simulink model "SMC_David_RedondoQuintero"  (R2023b)
settings: Solver=ode45  StartTime=0.0  StopTime=50  MaxStep=0.01  RelTol=1e-3
InitFcn:
  | R=2;
  | L=0.5;
  | Kb=0.01;
  | Ke=0.5;
  | Kt=0.5;
  | J=0.05;
undefined symbols (not defined in the file): sgn
libraries: simulink x3
settings Model: Creator=Usuario  LastModifiedBy=Usuario
settings SolverCC: ZeroCrossAlgorithm=Adaptive

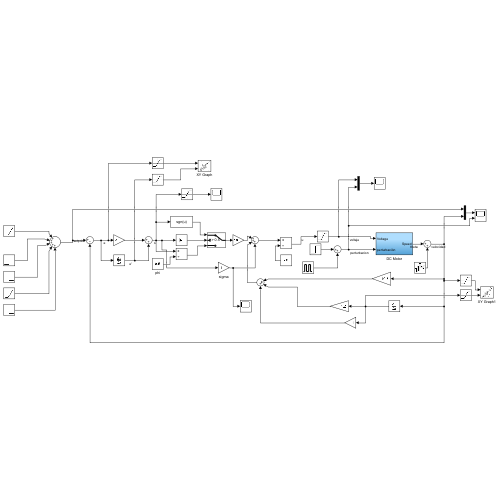
[thumbnail: Simulink's stored preview of the top-level diagram]
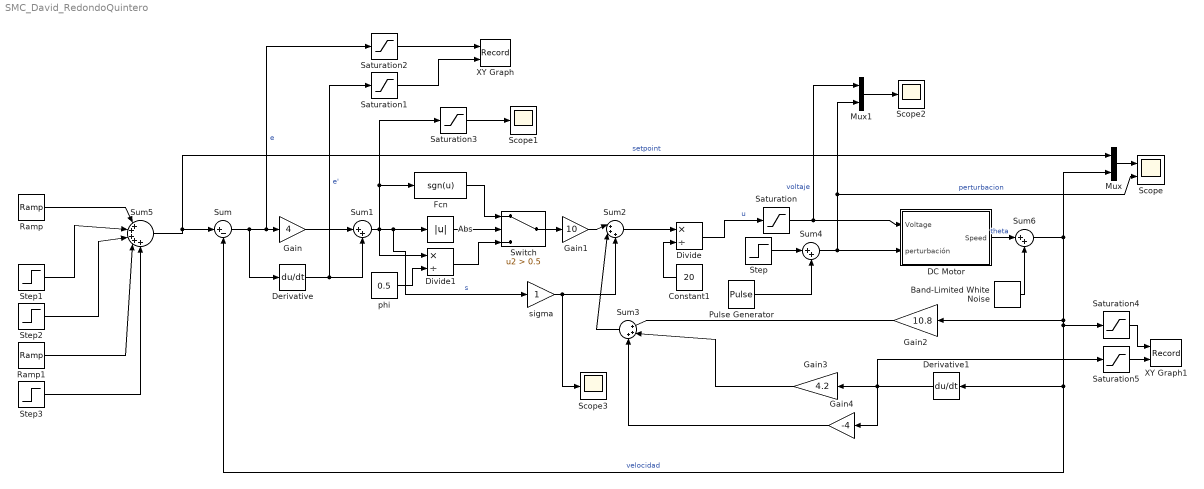
== system SMC_David_RedondoQuintero ==
  Abs : Abs  SaturateOnIntegerOverflow=off
  Band-Limited White Noise : simulink/Sources/Band-Limited White Noise  Cov=[0.0001]  Ts=0.1  seed=[23341]
  Constant1 : Constant  Value=20
  DC Motor : Subsystem
  Derivative : Derivative
  Derivative1 : Derivative
  Divide : Product  Inputs=*/
  Divide1 : Product  Inputs=*/
  Fcn : Fcn  Expr=sgn(u)
  Gain : Gain  Gain=4
  Gain1 : Gain  Gain=10
  Gain2 : Gain  Gain=10.8
  Gain3 : Gain  Gain=4.2
  Gain4 : Gain  Gain=-4
  Mux : Mux  Inputs=2
  Mux1 : Mux  Inputs=2
  Pulse Generator : DiscretePulseGenerator  PulseType=Time based  Amplitude=4  Period=10  PulseWidth=10  PhaseDelay=4
  Ramp : simulink/Sources/Ramp  slope=0.1  start=0  InitialOutput=0
  Ramp1 : simulink/Sources/Ramp  slope=-0.1  start=17  InitialOutput=0
  Saturation : Saturate  UpperLimit=12  LowerLimit=-12
  Saturation{1..5} (5 alike) : Saturate  UpperLimit=10  LowerLimit=-10
  Scope : Scope  NumInputPorts=2
  Scope1 : Scope
  Scope2 : Scope
  Scope3 : Scope
  Step : Step  Time=28  After=2  SampleTime=0
  Step1 : Step  Time=6  After=4  SampleTime=0
  Step2 : Step  Time=14  After=-2  SampleTime=0
  Step3 : Step  Time=19  After=-2  SampleTime=0
  Sum : Sum  Inputs=|+-
  Sum1 : Sum  Inputs=|++
  Sum2 : Sum  Inputs=|+++
  Sum3 : Sum  Inputs=|+++
  Sum4 : Sum  Inputs=|++
  Sum5 : Sum  Inputs=|+++++
  Sum6 : Sum  Inputs=|++
  Switch : Switch  Criteria=u2 > Threshold  Threshold=0.5  SaturateOnIntegerOverflow=off  InputSameDT=off
  XY Graph : Record  FileSettingsInternal="{\"entries\":[{\"content\":{\"excelSettings\":{\"content\":{},\"type\":\"Streamout.ExcelSettings\"}},\"type\":\"Streamout.FileSettingStorage\",\"uuid\":\"\"}],\"packageUris\":[\"http:\\/\\/schema.mathworks.com\\/mf0\\/streamout_blocks\\/R2020a\"],\"version\":\"1.0\"}"  Layout=[1 1]  SignalsInternal="{\"entries\":[{\"content\":{\"signals\":[{\"content\":{\"blockPath\":[],\"dimensions\":[1],\"domain\":\"\",\"lineColor\":\"#fe330a\",\"plots\":[1],\"port\":1,\"sid\":[\"\"],\"signalID\":13438,\"signalName\":\"Saturation2\"},\"type\":\"RecordBlkView.Signal\",\"uuid\":\"\"},{\"content\":{\"blockPath\":[],\"dimensions\":[1],\"domain\":\"\",\"lineColor\":\"#22b573\",\"plots\":[1],\"port\":2,\"sid\":[\"\"],\"signalID\":13442,\"signalName\":\"Saturation1\"},\"type\":\"RecordBlkView.Signal\",\"uuid\":\"\"}]},\"type\":\"RecordBlkView.InputSignals\",\"uuid\":\"\"}],\"packageUris\":[\"http:\\/\\/schema.mathworks.com\\/mf0\\/streamout_blocks\\/R2020a\"],\"version\":\"1.0\"}"  VisualizationBindings="{\"xyplotplugin\":{\"info\":[{\"series\":[{\"bindingParametersList\":[{\"parameter\":\"X-Axis\",\"signalID\":13438,\"signalName\":\"Saturation2\"},{\"parameter\":\"Y-Axis\",\"signalID\":13442,\"signalName\":\"Saturation1\"}],\"seriesID\":33756}],\"subplotID\":1}]}}"  CompatibilityTag=XY
  XY Graph1 : Record  FileSettingsInternal="{\"entries\":[{\"content\":{\"excelSettings\":{\"content\":{},\"type\":\"Streamout.ExcelSettings\"}},\"type\":\"Streamout.FileSettingStorage\",\"uuid\":\"\"}],\"packageUris\":[\"http:\\/\\/schema.mathworks.com\\/mf0\\/streamout_blocks\\/R2020a\"],\"version\":\"1.0\"}"  Layout=[1 1]  SignalsInternal="{\"entries\":[{\"content\":{\"signals\":[{\"content\":{\"blockPath\":[],\"dimensions\":[1],\"domain\":\"\",\"lineColor\":\"#0072bd\",\"plots\":[1],\"port\":1,\"sid\":[\"\"],\"signalID\":13446,\"signalName\":\"velocidad\"},\"type\":\"RecordBlkView.Signal\",\"uuid\":\"\"},{\"content\":{\"blockPath\":[],\"dimensions\":[1],\"domain\":\"\",\"lineColor\":\"#d95319\",\"plots\":[1],\"port\":2,\"sid\":[\"\"],\"signalID\":13450,\"signalName\":\"Derivative1\"},\"type\":\"RecordBlkView.Signal\",\"uuid\":\"\"}]},\"type\":\"RecordBlkView.InputSignals\",\"uuid\":\"\"}],\"packageUris\":[\"http:\\/\\/schema.mathworks.com\\/mf0\\/streamout_blocks\\/R2020a\"],\"version\":\"1.0\"}"  VisualizationBindings="{\"xyplotplugin\":{\"info\":[{\"series\":[{\"bindingParametersList\":[{\"parameter\":\"X-Axis\",\"signalID\":13446,\"signalName\":\"velocidad\"},{\"parameter\":\"Y-Axis\",\"signalID\":13450,\"signalName\":\"Derivative1\"}],\"seriesID\":6486}],\"subplotID\":1}]}}"  CompatibilityTag=XY
  phi : Constant  Value=0.5
  sigma : Gain
  wires:
  Divide1/1 -> Switch/3
  DC Motor/1(Speed) -> Sum6/1  "theta"
  Sum5/1 -> Mux/1, Sum/1  "setpoint"
  Divide/1 -> Saturation/1  "u"
  Sum1/1 -> Divide1/1, Fcn/1, Saturation3/1, sigma/1, Abs/1  "s"
  Constant1/1 -> Divide/2
  Mux/1 -> Scope/1
  Sum2/1 -> Divide/1
  Derivative1/1 -> Gain4/1, Saturation5/1, Gain3/1
  Abs/1 -> Switch/2
  Gain4/1 -> Sum3/3
  Gain/1 -> Sum1/1
  Gain2/1 -> Sum3/1
  phi/1 -> Divide1/2
  Derivative/1 -> Saturation1/1, Sum1/2  "e'"
  Sum/1 -> Derivative/1, Saturation2/1, Gain/1  "e"
  Gain1/1 -> Sum2/1
  Switch/1 -> Gain1/1
  Fcn/1 -> Switch/1
  Sum4/1 -> Mux1/2, Scope/2, DC Motor/2(perturbación)  "perturbacion"
  Step2/1 -> Sum5/3
  Step1/1 -> Sum5/2
  Ramp/1 -> Sum5/1
  Ramp1/1 -> Sum5/4
  Step3/1 -> Sum5/5
  Sum6/1 -> Sum/2, Derivative1/1, Saturation4/1, Gain2/1, Mux/2  "velocidad"
  Sum3/1 -> Sum2/2
  sigma/1 -> Sum2/3, Scope3/1
  Step/1 -> Sum4/1
  Pulse Generator/1 -> Sum4/2
  Saturation1/1 -> XY Graph/2
  Saturation2/1 -> XY Graph/1
  Saturation3/1 -> Scope1/1
  Mux1/1 -> Scope2/1
  Band-Limited White Noise/1 -> Sum6/2
  Saturation/1 -> Mux1/1, DC Motor/1(Voltage)  "voltaje"
  Gain3/1 -> Sum3/2
  Saturation4/1 -> XY Graph1/1
  Saturation5/1 -> XY Graph1/2

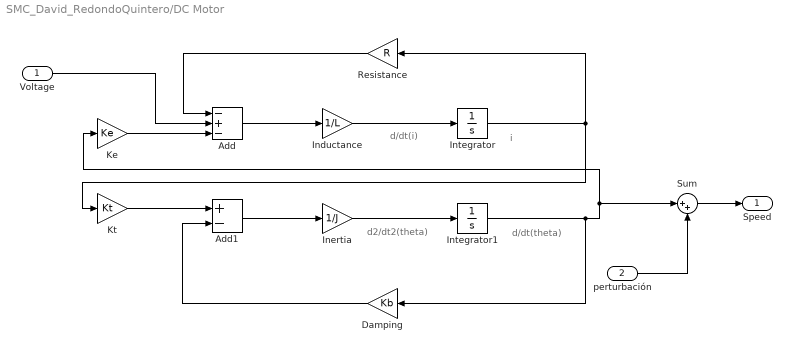
== system SMC_David_RedondoQuintero/DC Motor ==
  note: i
  note: d/dt(i)
  note: d/dt(theta)
  note: d2/dt2(theta)
  Voltage : Inport
  perturbación : Inport  Port=2
  Add : Sum  Inputs=-+-
  Add1 : Sum  Inputs=+-
  Damping : Gain  Gain=Kb
  Inductance : Gain  Gain=1/L
  Inertia : Gain  Gain=1/J
  Integrator : Integrator
  Integrator1 : Integrator
  Ke : Gain  Gain=Ke
  Kt : Gain  Gain=Kt
  Resistance : Gain  Gain=R
  Sum : Sum  Inputs=|++
  Speed : Outport
  wires:
  Inductance/1 -> Integrator/1
  Integrator1/1 -> Damping/1, Ke/1, Sum/1
  Inertia/1 -> Integrator1/1
  Kt/1 -> Add1/1
  Voltage/1 -> Add/2
  Resistance/1 -> Add/1
  Damping/1 -> Add1/2
  Ke/1 -> Add/3
  Add/1 -> Inductance/1
  Add1/1 -> Inertia/1
  Sum/1 -> Speed/1
  perturbación/1 -> Sum/2
  Integrator/1 -> Resistance/1, Kt/1
